simulink model "hcc_sm_v6_circuit2"  (R2024b)
settings: Solver=VariableStepAuto  StartTime=0.0  StopTime=0.2  RelTol=1e-3
libraries: spsSeriesRLCBranchLib x530, spsGtoLib x144, spsDiodeLib x78, spsVoltageMeasurementLib x6, spsGroundLib x2, spsDCVoltageSourceLib x1, spsNonlinearResistorLib x1, spsThreePhaseTransformerTwoWindingsLib x1, spsThreePhaseSourceLib x1, spspowerguiLib x1
(part 3 of 3)

== system hcc_sm_v6_circuit2/Bridge5/Segment4/SaturableReactor ==
  note: C
  Cs : spsSeriesRLCBranchLib/Series RLC Branch  LConnTagsString=__new0  RConnTagsString=__new0  BranchType=C  Resistance=88  Inductance=6.3e-6  SetiL0=off  InitialCurrent=0  Capacitance=250e-12  Setx0=off  InitialVoltage=0  Measurements=None
  LAir : spsSeriesRLCBranchLib/Series RLC Branch  LConnTagsString=__new0  RConnTagsString=__new0  BranchType=L  Resistance=88  Inductance=6.3e-6  SetiL0=off  InitialCurrent=0  Capacitance=2.62e-06  Setx0=off  InitialVoltage=0  Measurements=None
  Lm : spsSeriesRLCBranchLib/Series RLC Branch  LConnTagsString=__new0  RConnTagsString=__new0  BranchType=L  Resistance=88  Inductance=524.8e-6  SetiL0=off  InitialCurrent=0  Capacitance=2.62e-06  Setx0=off  InitialVoltage=0  Measurements=None
  Re : spsSeriesRLCBranchLib/Series RLC Branch  LConnTagsString=__new0  RConnTagsString=__new0  BranchType=R  Resistance=250  Inductance=6.3e-6  SetiL0=off  InitialCurrent=0  Capacitance=2.62e-06  Setx0=off  InitialVoltage=0  Measurements=None
  A : PMIOPort  Side=Left
  B : PMIOPort  Port=2  Side=Right
  connections:
  B/RConn1 -- Re/RConn1 -- Lm/RConn1 -- Cs/RConn1
  Lm/LConn1 -- Re/LConn1 -- LAir/RConn1
  LAir/LConn1 -- Cs/LConn1 -- A/RConn1

== system hcc_sm_v6_circuit2/Bridge6/Segment1/SaturableReactor ==
  note: C
  Cs : spsSeriesRLCBranchLib/Series RLC Branch  LConnTagsString=__new0  RConnTagsString=__new0  BranchType=C  Resistance=88  Inductance=6.3e-6  SetiL0=off  InitialCurrent=0  Capacitance=250e-12  Setx0=off  InitialVoltage=0  Measurements=None
  LAir : spsSeriesRLCBranchLib/Series RLC Branch  LConnTagsString=__new0  RConnTagsString=__new0  BranchType=L  Resistance=88  Inductance=6.3e-6  SetiL0=off  InitialCurrent=0  Capacitance=2.62e-06  Setx0=off  InitialVoltage=0  Measurements=None
  Lm : spsSeriesRLCBranchLib/Series RLC Branch  LConnTagsString=__new0  RConnTagsString=__new0  BranchType=L  Resistance=88  Inductance=524.8e-6  SetiL0=off  InitialCurrent=0  Capacitance=2.62e-06  Setx0=off  InitialVoltage=0  Measurements=None
  Re : spsSeriesRLCBranchLib/Series RLC Branch  LConnTagsString=__new0  RConnTagsString=__new0  BranchType=R  Resistance=250  Inductance=6.3e-6  SetiL0=off  InitialCurrent=0  Capacitance=2.62e-06  Setx0=off  InitialVoltage=0  Measurements=None
  A : PMIOPort  Side=Left
  B : PMIOPort  Port=2  Side=Right
  connections:
  A/RConn1 -- Cs/LConn1 -- LAir/LConn1
  LAir/RConn1 -- Re/LConn1 -- Lm/LConn1
  Cs/RConn1 -- Lm/RConn1 -- Re/RConn1 -- B/RConn1

== system hcc_sm_v6_circuit2/Bridge6/Segment2/SaturableReactor ==
  note: C
  Cs : spsSeriesRLCBranchLib/Series RLC Branch  LConnTagsString=__new0  RConnTagsString=__new0  BranchType=C  Resistance=88  Inductance=6.3e-6  SetiL0=off  InitialCurrent=0  Capacitance=250e-12  Setx0=off  InitialVoltage=0  Measurements=None
  LAir : spsSeriesRLCBranchLib/Series RLC Branch  LConnTagsString=__new0  RConnTagsString=__new0  BranchType=L  Resistance=88  Inductance=6.3e-6  SetiL0=off  InitialCurrent=0  Capacitance=2.62e-06  Setx0=off  InitialVoltage=0  Measurements=None
  Lm : spsSeriesRLCBranchLib/Series RLC Branch  LConnTagsString=__new0  RConnTagsString=__new0  BranchType=L  Resistance=88  Inductance=524.8e-6  SetiL0=off  InitialCurrent=0  Capacitance=2.62e-06  Setx0=off  InitialVoltage=0  Measurements=None
  Re : spsSeriesRLCBranchLib/Series RLC Branch  LConnTagsString=__new0  RConnTagsString=__new0  BranchType=R  Resistance=250  Inductance=6.3e-6  SetiL0=off  InitialCurrent=0  Capacitance=2.62e-06  Setx0=off  InitialVoltage=0  Measurements=None
  A : PMIOPort  Side=Left
  B : PMIOPort  Port=2  Side=Right
  connections:
  B/RConn1 -- Re/RConn1 -- Lm/RConn1 -- Cs/RConn1
  Lm/LConn1 -- Re/LConn1 -- LAir/RConn1
  LAir/LConn1 -- Cs/LConn1 -- A/RConn1

== system hcc_sm_v6_circuit2/Bridge6/Segment3/SaturableReactor ==
  note: C
  Cs : spsSeriesRLCBranchLib/Series RLC Branch  LConnTagsString=__new0  RConnTagsString=__new0  BranchType=C  Resistance=88  Inductance=6.3e-6  SetiL0=off  InitialCurrent=0  Capacitance=250e-12  Setx0=off  InitialVoltage=0  Measurements=None
  LAir : spsSeriesRLCBranchLib/Series RLC Branch  LConnTagsString=__new0  RConnTagsString=__new0  BranchType=L  Resistance=88  Inductance=6.3e-6  SetiL0=off  InitialCurrent=0  Capacitance=2.62e-06  Setx0=off  InitialVoltage=0  Measurements=None
  Lm : spsSeriesRLCBranchLib/Series RLC Branch  LConnTagsString=__new0  RConnTagsString=__new0  BranchType=L  Resistance=88  Inductance=524.8e-6  SetiL0=off  InitialCurrent=0  Capacitance=2.62e-06  Setx0=off  InitialVoltage=0  Measurements=None
  Re : spsSeriesRLCBranchLib/Series RLC Branch  LConnTagsString=__new0  RConnTagsString=__new0  BranchType=R  Resistance=250  Inductance=6.3e-6  SetiL0=off  InitialCurrent=0  Capacitance=2.62e-06  Setx0=off  InitialVoltage=0  Measurements=None
  A : PMIOPort  Side=Left
  B : PMIOPort  Port=2  Side=Right
  connections:
  A/RConn1 -- Cs/LConn1 -- LAir/LConn1
  LAir/RConn1 -- Re/LConn1 -- Lm/LConn1
  Cs/RConn1 -- Lm/RConn1 -- Re/RConn1 -- B/RConn1

== system hcc_sm_v6_circuit2/Bridge6/Segment4/SaturableReactor ==
  note: C
  Cs : spsSeriesRLCBranchLib/Series RLC Branch  LConnTagsString=__new0  RConnTagsString=__new0  BranchType=C  Resistance=88  Inductance=6.3e-6  SetiL0=off  InitialCurrent=0  Capacitance=250e-12  Setx0=off  InitialVoltage=0  Measurements=None
  LAir : spsSeriesRLCBranchLib/Series RLC Branch  LConnTagsString=__new0  RConnTagsString=__new0  BranchType=L  Resistance=88  Inductance=6.3e-6  SetiL0=off  InitialCurrent=0  Capacitance=2.62e-06  Setx0=off  InitialVoltage=0  Measurements=None
  Lm : spsSeriesRLCBranchLib/Series RLC Branch  LConnTagsString=__new0  RConnTagsString=__new0  BranchType=L  Resistance=88  Inductance=524.8e-6  SetiL0=off  InitialCurrent=0  Capacitance=2.62e-06  Setx0=off  InitialVoltage=0  Measurements=None
  Re : spsSeriesRLCBranchLib/Series RLC Branch  LConnTagsString=__new0  RConnTagsString=__new0  BranchType=R  Resistance=250  Inductance=6.3e-6  SetiL0=off  InitialCurrent=0  Capacitance=2.62e-06  Setx0=off  InitialVoltage=0  Measurements=None
  A : PMIOPort  Side=Left
  B : PMIOPort  Port=2  Side=Right
  connections:
  B/RConn1 -- Re/RConn1 -- Lm/RConn1 -- Cs/RConn1
  Lm/LConn1 -- Re/LConn1 -- LAir/RConn1
  LAir/LConn1 -- Cs/LConn1 -- A/RConn1
